simulink model "telemetrySources"  (Simulink 6.6)
settings: Solver=ode3  StartTime=0.0  StopTime=time(end)  FixedStep=0.01  RelTol=1e-3
undefined symbols (not defined in the file or in its folder): ACC_hil, baroMeanTemp, baroOffset, baroScale, baroTempK, baseHeight, baseTemp, DYN_hil, gaind, GS_location, ISA_rho0, lapseRate, MAG_hil, magMeanTemp, magOffset, magScale, magTempK, param_acc, param_mag, pitMeanTemp, pitotOffset, pitotScale, pitTempK, polesd, STA_hil, T, TEM_hil, zerosd
libraries: simulink x6, SLUGS_Library x6, aerolibconvert2 x1
(part 2 of 2)

== matlab function Accceleration/3D LowPass/myMux Fun1 ==
  data: u1 input inherited; y output inherited; u2 input inherited; u3 input inherited
function y = myMux(u1, u2, u3)
% This block supports an embeddable subset of the MATLAB language.
% See the help menu for details. 

y = [u1(1); u2(1); u3(1)];

== matlab function Static/Baro Altimeter/Enables/Disables the Computation of initial Baro Bias ==
  data: tOut output inherited
function tOut = getTIni

persistent aveCount;
persistent tIni;

if isempty(aveCount)
    aveCount =1;
    tIni = 1;
end;

if aveCount < 2500
    aveCount = aveCount + 1;
end

if aveCount == 2500
    tIni =0;
    aveCount = aveCount + 1;
end

tOut = tIni;

%if aveCount > 500
%    tIni = 0;
%end

% if isempty(aveCount)
%     aveCount =1;
%     initBias = [0.0 0.0 0.0]';
% end;
%     
% if (aveCount<10)
%     initBias = initBias+ Raw;
%     bias = initBias/aveCount;
%     aveCount = aveCount +1;
% end;
% 
% if (aveCount == 10)
%     initBias = initBias/(aveCount-1);
%     aveCount = 100;
% end;
% 
% if (aveCount == 100)
%     bias = initBias;
% end;
